simulink model "project1_2023a"  (R2021b)
settings: Solver=ode2  StartTime=0.0  StopTime=600  FixedStep=1  MaxStep=0.2  MinStep=1e-20  RelTol=1e-3
values from neighbouring files (symbols this model uses):
  A_F = 1.93    [init.m]
  C_0 = 0.015    [init.m]
  C_D = 0.35    [init.m]
  E_ess_max = E_batt_kW * 1000 * 3600    (= 7200000)    [init.m]
  eta_ess = 0.8    [init.m]
  g = 9.81    [init.m]
  G_diff = 0.268    [init.m]
  G_elec = 1    [init.m]
  grams_per_hr_to_gal_per_s = 9.778e-8    (= 9.778e-08)    [init.m]
  M_veh = M_glider + M_passengers + M_batt    (= 1976)    [init.m]
  meters_to_mi = 1/1609    (= 0.000621504039776)    [init.m]
  mi_per_hr_to_m_per_s = 0.44704    [init.m]
  r_wheel = 0.2794    [init.m]
  rho = 1.225    [init.m]
  SOC_init = 0.5    [init.m]
undefined symbols (not defined in the file or in its folder): eng_map, param, udds
settings Model: Creator=wasynczu  LastModifiedBy=Arijeet
settings SolverCC: AlgebraicLoopSolver=TrustRegion
settings DebuggingCC: SFMachineParentedDataDiag=warning

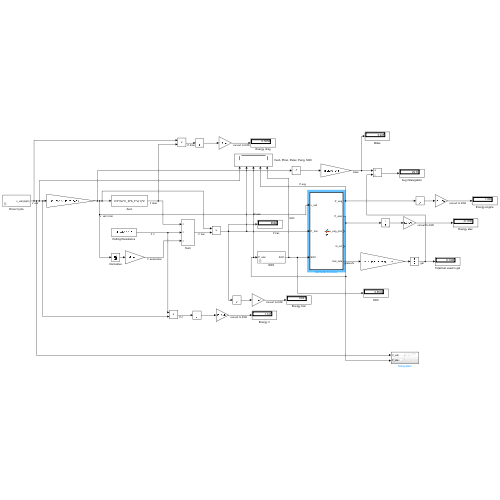
[thumbnail: Simulink's stored preview of the top-level diagram]
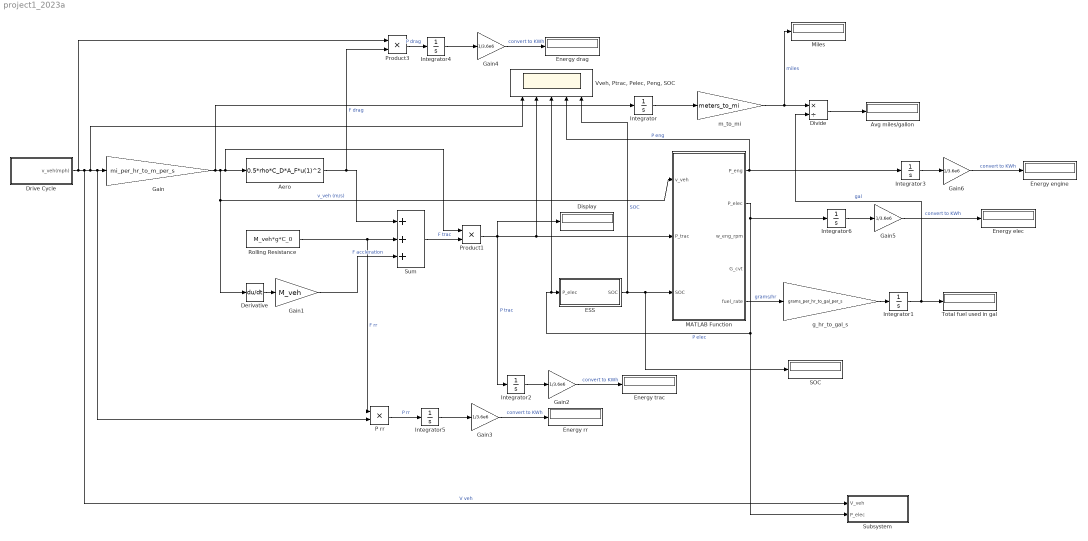
== system project1_2023a ==
  Aero : Fcn  Expr=0.5*rho*C_D*A_F*u(1)^2
  Avg miles/gallon : Display
  Derivative : Derivative
  Display : Display
  Divide : Product  Inputs=*/
  Drive Cycle : Subsystem  mask{schedule=udds}
      mask prompts: schedule "drive schedule"
      mask init:
      | N=length(schedule(:,1));
  ESS : Subsystem  mask{E_max=E_ess_max, eta_ess=eta_ess}
      mask prompts: E_max "Maximum energy, J"; eta_ess "round-trip efficiency"
  Energy drag : Display
  Energy elec : Display
  Energy engine : Display
  Energy rr : Display
  Energy trac : Display
  Gain : Gain  Gain=mi_per_hr_to_m_per_s
  Gain1 : Gain  Gain=M_veh
  Gain{2..6} (5 alike) : Gain  Gain=1/3.6e6
  Integrator{,1..6} (7 alike) : Integrator
  MATLAB Function : MATLAB Function  TreatAsAtomicUnit=on
  Miles : Display
  P rr : Product
  Product1 : Product
  Product3 : Product
  Rolling Resistance : Constant  Value=M_veh*g*C_0
  SOC : Display
  Subsystem : Subsystem
  Sum : Sum  Inputs=+++
  Total fuel used in gal : Display
  "Vveh, Ptrac, Pelec, Peng, SOC" : Scope  NumInputPorts=5
  g_hr_to_gal_s : Gain  Gain=grams_per_hr_to_gal_per_s
  m_to_mi : Gain  Gain=meters_to_mi
  wires:
  Drive Cycle/1(v_veh(mph)) -> Product3/1, "Vveh, Ptrac, Pelec, Peng, SOC"/1, P rr/2, Gain/1, Subsystem/1(V_veh)  "V veh"
  Gain/1 -> Integrator/1, Derivative/1, MATLAB Function/1(v_veh), Product1/1, Aero/1  "v_veh (m/s)"
  Derivative/1 -> Gain1/1
  Aero/1 -> Product3/2, Sum/1  "F drag"
  Rolling Resistance/1 -> Sum/2, P rr/1  "F rr"
  Gain1/1 -> Sum/3  "F accleration"
  Sum/1 -> Product1/2  "F trac"
  Product1/1 -> Integrator2/1, MATLAB Function/2(P_trac), "Vveh, Ptrac, Pelec, Peng, SOC"/2, Display/1  "P trac"
  MATLAB Function/2(P_elec) -> Integrator6/1, Subsystem/2(P_elec), "Vveh, Ptrac, Pelec, Peng, SOC"/3, ESS/1(P_elec)  "P elec"
  ESS/1(SOC) -> SOC/1, MATLAB Function/3(SOC), "Vveh, Ptrac, Pelec, Peng, SOC"/5  "SOC"
  MATLAB Function/5(fuel_rate) -> g_hr_to_gal_s/1  "grams/hr"
  MATLAB Function/1(P_eng) -> Integrator3/1, "Vveh, Ptrac, Pelec, Peng, SOC"/4  "P eng"
  g_hr_to_gal_s/1 -> Integrator1/1
  Integrator1/1 -> Divide/2, Total fuel used in gal/1  "gal"
  Integrator/1 -> m_to_mi/1
  m_to_mi/1 -> Miles/1, Divide/1  "miles"
  Divide/1 -> Avg miles/gallon/1
  Product3/1 -> Integrator4/1  "P drag"
  P rr/1 -> Integrator5/1  "P rr"
  Integrator3/1 -> Gain6/1
  Gain6/1 -> Energy engine/1  "convert to KWh"
  Integrator2/1 -> Gain2/1
  Gain2/1 -> Energy trac/1  "convert to KWh"
  Integrator5/1 -> Gain3/1
  Gain3/1 -> Energy rr/1  "convert to KWh"
  Integrator4/1 -> Gain4/1
  Gain4/1 -> Energy drag/1  "convert to KWh"
  Integrator6/1 -> Gain5/1
  Gain5/1 -> Energy elec/1  "convert to KWh"

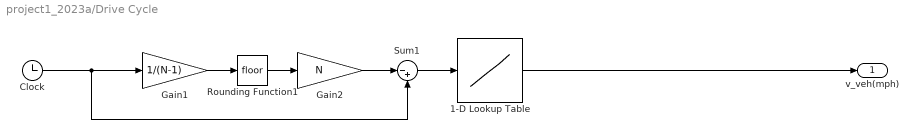
== system project1_2023a/Drive Cycle ==
  1-D Lookup Table : Lookup_n-D  NumberOfTableDimensions=1  BreakpointsForDimension1=schedule(:,1)  Table=schedule(:,2)  InterpMethod=Cubic spline  InternalRulePriority=Speed  RndMeth=Simplest  InputSameDT=on
  Clock : Clock
  Gain1 : Gain  Gain=1/(N-1)
  Gain2 : Gain  Gain=N
  Rounding Function1 : Rounding
  Sum1 : Sum  Inputs=|-+
  v_veh(mph) : Outport  VectorParamsAs1DForOutWhenUnconnected=off
  wires:
  Clock/1 -> Gain1/1, Sum1/2
  Sum1/1 -> 1-D Lookup Table/1
  Gain2/1 -> Sum1/1
  Rounding Function1/1 -> Gain2/1
  Gain1/1 -> Rounding Function1/1
  1-D Lookup Table/1 -> v_veh(mph)/1

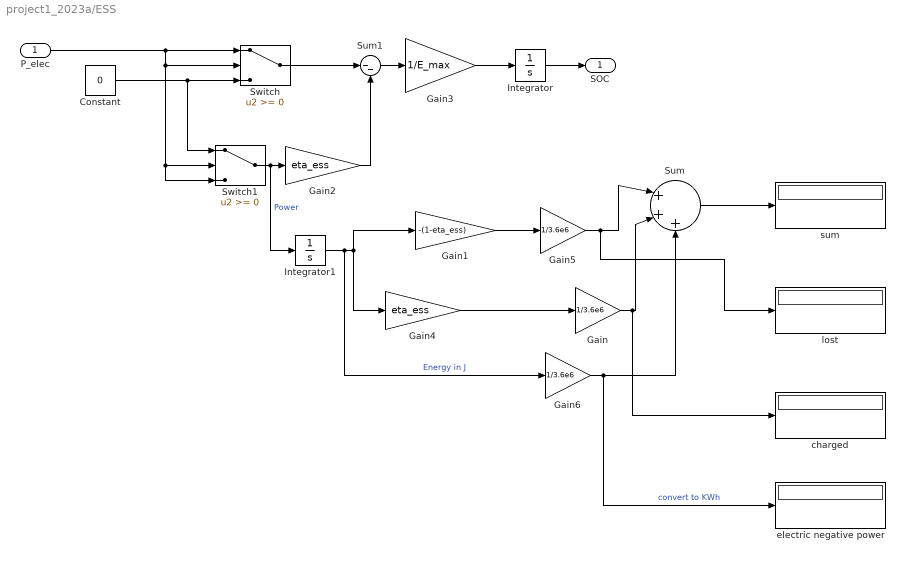
== system project1_2023a/ESS ==
  P_elec : Inport
  Constant : Constant  Value=0
  Gain : Gain  Gain=1/3.6e6
  Gain1 : Gain  Gain=-(1-eta_ess)
  Gain2 : Gain  Gain=eta_ess
  Gain3 : Gain  Gain=1/E_max  OutDataTypeStr=fixdt('double', 'DataTypeOverride', 'Off')
  Gain4 : Gain  Gain=eta_ess
  Gain5 : Gain  Gain=1/3.6e6
  Gain6 : Gain  Gain=1/3.6e6
  Integrator : Integrator  InitialCondition=SOC_init  LimitOutput=on  UpperSaturationLimit=1  LowerSaturationLimit=0
  Integrator1 : Integrator
  Sum : Sum  Inputs=|+++
  Sum1 : Sum  Inputs=|--
  Switch : Switch  OutDataTypeStr=double
  Switch1 : Switch  OutDataTypeStr=double
  charged : Display
  electric negative power : Display
  lost : Display
  sum : Display
  SOC : Outport  VectorParamsAs1DForOutWhenUnconnected=off
  wires:
  P_elec/1 -> Switch1/2, Switch1/3, Switch/2, Switch/1
  Gain3/1 -> Integrator/1
  Gain2/1 -> Sum1/2
  Switch1/1 -> Integrator1/1, Gain2/1  "Power"
  Sum1/1 -> Gain3/1
  Switch/1 -> Sum1/1
  Constant/1 -> Switch1/1, Switch/3
  Integrator/1 -> SOC/1
  Integrator1/1 -> Gain6/1, Gain4/1, Gain1/1  "Energy in J"
  Gain4/1 -> Gain/1
  Gain1/1 -> Gain5/1
  Sum/1 -> sum/1
  Gain5/1 -> lost/1, Sum/1
  Gain6/1 -> electric negative power/1, Sum/3  "convert to KWh"
  Gain/1 -> charged/1, Sum/2

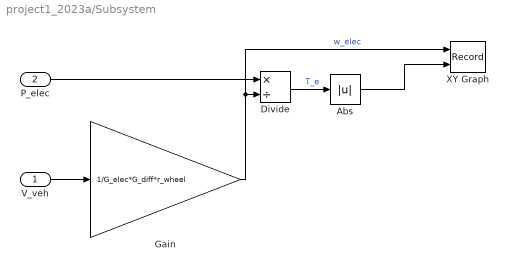
== system project1_2023a/Subsystem ==
  V_veh : Inport
  P_elec : Inport  Port=2
  Abs : Abs
  Divide : Product  Inputs=*/
  Gain : Gain  Gain=1/G_elec*G_diff*r_wheel
  XY Graph : Record  FileSettingsInternal="{\"entries\":[{\"content\":{\"excelSettings\":{\"content\":{},\"type\":\"Streamout.ExcelSettings\"}},\"type\":\"Streamout.FileSettingStorage\",\"uuid\":\"962208de-257e-4186-9ef0-22c69d48dc69\"}],\"packageUris\":[\"http://schema.mathworks.com/mf0/streamout_blocks/R2020a\"],\"version\":\"1.0\"}"  Layout=[1 1]  SignalsInternal="{\"entries\":[{\"content\":{\"signals\":[{\"content\":{\"blockPath\":[\"project1_2020a/Subsystem/XY Graph\"],\"channel\":[],\"dimensions\":[1],\"domain\":\"project1_2020a/Subsystem/XY Graph\",\"lineColor\":\"#a2142f\",\"plots\":[1],\"port\":1,\"sid\":[\"\"],\"signalID\":20,\"signalName\":\"w_elec\"},\"type\":\"RecordBlkView.Signal\",\"uuid\":\"3ecef69e-d5d6-4f59-a9d9-4f1274878a7e\"},{\"content\":{\"blockPath\":[\"project1_2020a/Subsystem/XY Graph\"],\"channel\":[],\"dimensions\":[1],\"domain\":\"project1_2020a/Subsystem/XY Graph\",\"lineColor\":\"#139fff\",\"plots\":[1],\"port\":2,\"sid\":[\"\"],\"signalID\":24,\"signalName\":\"Abs\"},\"type\":\"RecordBlkView.Signal\",\"uuid\":\"35bc9ded-e819-4871-ba10-393c62ec3042\"}]},\"type\":\"RecordBlkView.InputSignals\",\"uuid\":\"158c8ee5-9b3e-417e-bde7-377cada1a96d\"}],\"packageUris\":[\"http://schema.mathworks.com/mf0/streamout_blocks/R2020a\"],\"version\":\"1.0\"}"  VisualizationBindings="{\"xyplotplugin\":{\"info\":[{\"series\":[{\"bindingParametersList\":[{\"parameter\":\"X-Axis\",\"signalID\":20,\"signalName\":\"w_elec\"},{\"parameter\":\"Y-Axis\",\"signalID\":24,\"signalName\":\"Abs\"}],\"seriesID\":7640}],\"subplotID\":1}]}}"  CompatibilityTag=XY
  wires:
  V_veh/1 -> Gain/1
  Gain/1 -> XY Graph/1, Divide/2  "w_elec"
  P_elec/1 -> Divide/1
  Divide/1 -> Abs/1  "T_e"
  Abs/1 -> XY Graph/2

== matlab function project1_2023a/MATLAB Function ==
  data: v_veh input; P_eng output; P_trac input; SOC input; P_elec output; w_eng_rpm output; G_cvt output; fuel_rate output; param parameter; eng_map parameter
function [P_eng, P_elec, w_eng_rpm, G_cvt, fuel_rate] = fcn(v_veh, P_trac, SOC, param, eng_map)
%function [P_eng, P_elec, w_eng_rpm, G_cvt, fuel_rate] = fcn(v_veh, P_trac, SOC, param, eng_map)
%function [P_eng, P_elec, w_eng_rpm, G_cvt, fuel_rate] = fcn(v_veh, P_trac, SOC, param, eng_map)
%#codegen
%inputs:
    % v_veh, m/s
    % P_trac, W
    % SOC
    % param, structure of parameters
    % eng_map

% outputs:
    %   P_gen, P_elec in W
    %   w_eng_rpm, rpm
    %   G_cvt (cvt ratio)
    %   Fuel rate, grams/hr

v_veh_min = param.v_veh_min;    % minimum vehicle speed for engine to stay engaged, in m/s
P_eng_min = param.P_eng_min;    % minimum engine power in W
P_eng_max = param.P_eng_max ;   % maximum engine power
G_cvt_min = param.G_cvt_min;    % minimum cvt  ratio
G_diff = param.G_diff;          % differential gear ratio
r_wheel = param.r_wheel;        % wheel radius in m

if (v_veh < v_veh_min)  % disengage clutch, idle engine, electric propulsion
   P_elec = P_trac;
   P_eng = 0;
   fuel_rate = 0; % g/hr;
   w_eng_rpm = 1000; % rpm
   G_cvt = G_cvt_min;
   return  
end

% if here, v_veh > v_veh_min
if(P_trac < P_eng_min)   % clutch engaged but engine idling
   P_elec = P_trac;
   fuel_rate = 0;
   P_eng = 0;
   w_eng_rpm =  1000; % rpm
   w_eng = w_eng_rpm * pi / 30; % rad/s
   % set G_cvt so engine speed is 1000 rpm
   G_cvt = v_veh/G_diff/w_eng/r_wheel;
   return     
end

if(P_trac > P_eng_max) % high-speed boost
   P_elec = P_trac - P_eng_max;
   P_eng = P_eng_max;
   bsfc = interp1(eng_map(:,2), eng_map(:,3), P_eng/1000, 'pchip', 'extrap');
   fuel_rate = bsfc*P_eng/1000; % grams/hr
   w_eng_rpm = interp1(eng_map(:,2), eng_map(:,1), P_eng/1000, 'pchip', 'extrap');
   w_eng = w_eng_rpm * pi / 30; % convert to rad/s
   G_cvt =  v_veh/r_wheel/G_diff/w_eng; % required CVT ratio
   return   
end

% if here, v_veh > v_veh_min and P_eng_min < P_trac < P_eng_max
% try to get SOC back to 0.5

P_elec = 20000*(SOC - 0.5); 
if(P_elec > 4000)
    P_elec = 4000;
end
if(P_elec < -4000)
    P_elec = -4000;
end

P_eng = P_trac - P_elec;


if(P_eng < P_eng_min) 
   % clutch engaged, but no fuel
   P_eng = 0;
   P_elec = P_trac;
   fuel_rate = 0;
   w_eng_rpm = 1000;
   w_eng = w_eng_rpm * 2 * pi / 60; % in rad/s
   % set G_cvt so engine speed is 1000 rpm
   G_cvt = v_veh/G_diff/w_eng/r_wheel;
   return
end

if(P_eng > P_eng_max)
    P_eng = P_eng_max;
    P_elec = P_trac - P_eng_max;
end

bsfc = interp1(eng_map(:,2), eng_map(:,3), P_eng/1000, 'pchip', 'extrap');
fuel_rate = bsfc*P_eng/1000; % grams/hr

w_eng_rpm = interp1(eng_map(:,2), eng_map(:,1), P_eng/1000, 'pchip', 'extrap');
if(w_eng_rpm < 1000)
    w_eng_rpm = 1000;
end
w_eng = w_eng_rpm * pi / 30;  % convert to rad/s
G_cvt =  v_veh/r_wheel/G_diff/w_eng;

if (G_cvt < G_cvt_min) % set G_cvt = G_cvt_min, recalculate w_eng, P_eng, and P_elec
   G_cvt = G_cvt_min;
   w_eng = v_veh/G_diff/r_wheel/G_cvt;
   w_eng_rpm = w_eng*30/pi;  % in rpm
   P_eng = 1000*interp1(eng_map(:,1), eng_map(:,2), w_eng, 'pchip', 'extrap'); % in W
   if(P_eng < 0)
       P_eng = 0;
   end
   P_elec = P_trac - P_eng;
   bsfc = interp1(eng_map(:,1), eng_map(:,3), w_eng, 'pchip', 'extrap');
   fuel_rate = bsfc*P_eng/1000; % grams/hr
 end
